simulink model "ExecutionTiming"  (R2014b)
settings: Solver=ode3  StartTime=0.0  StopTime=60  RelTol=1e-3
libraries: LegIK x6, BeagleBoneBlackCom x2, ServoCommand x2, MainController x1, Coord_BodyToLeg x1, TriggerSystem x1
settings Model: SimulationMode=processor-in-the-loop (pil)  Creator=dan  LastModifiedBy=Sebastian
settings SolverCC: InsertRTBMode=Never (minimum delay)
settings DataIOCC: SaveOutput=off  InspectSignalLogs=on  SaveTime=off
settings OptimizationCC: ExpressionDepthLimit=2147483647  OptimizeModelRefInitCode=on  LifeSpan=1  MaxStackSize=64
settings DebuggingCC: UnderspecifiedInitializationDetection=Classic  MergeDetectMultiDrivingBlocksExec=none  SignalResolutionControl=TryResolveAllWithWarning  MultiTaskDSMMsg=warning  MultiTaskCondExecSysMsg=none  ParameterPrecisionLossMsg=none  FcnCallInpInsideContextMsg=UseLocalSettings  UnconnectedInputMsg=none  UnconnectedOutputMsg=none  StateNameClashWarn=warning
settings HardwareCC: ProdLargestAtomicInteger=Long  ProdLargestAtomicFloat=Double  ProdEndianess=LittleEndian  ProdHWDeviceType=ARM Compatible->ARM Cortex  TargetBitPerChar=16  TargetBitPerInt=16  TargetBitPerPointer=16  TargetLargestAtomicInteger=Integer  TargetIntDivRoundTo=Zero  TargetEndianess=LittleEndian  TargetWordSize=16  TargetHWDeviceType=Texas Instruments->C2000
settings RTWCC: SystemTargetFile=ert.tlc  TemplateMakefile=ert_default_tmf  Description=Embedded Coder  ProcessScript=ert_make_rtw_hook  Toolchain=Linaro Toolchain v4.8  BuildConfiguration=Specify  CodeExecutionProfiling=on  CodeExecutionProfileVariable=executionProfile99  CodeProfilingSaveOptions=AllData  IncludeERTFirstTime=on
settings CodeAppCC: IgnoreCustomStorageClasses=off  CustomSymbolStrType=$N$R$M  InternalIdentifier=Classic
settings ERTTargetCC: CodeReplacementLibrary=ARM Cortex-A  MatFileLogging=on  SupportNonInlinedSFcns=on  SupportVariableSizeSignals=on

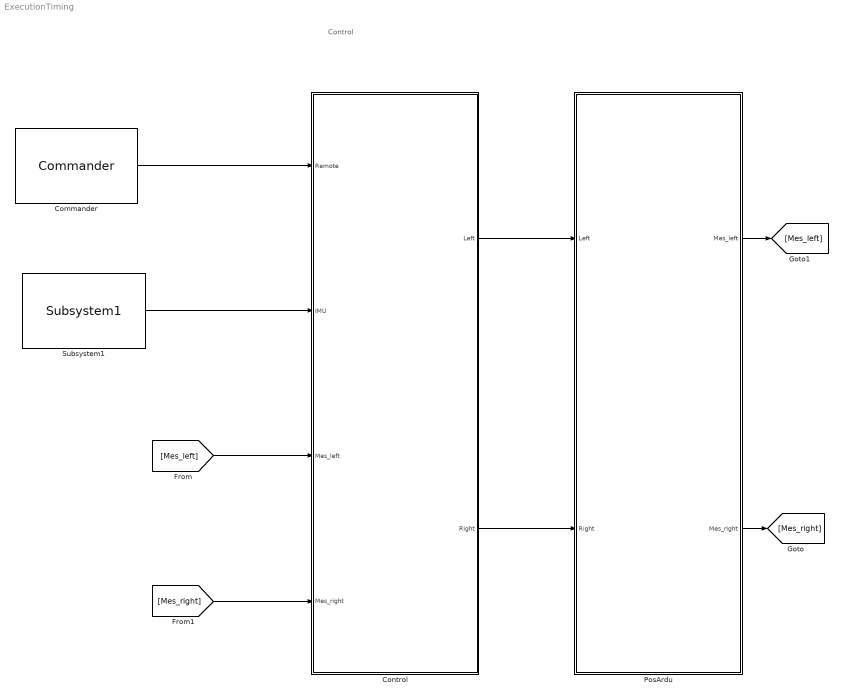
== system ExecutionTiming ==
  note: Control
  Commander : BeagleBoneBlackCom/Commander  portNbr=Uart 2
  Control : Subsystem  TreatAsAtomicUnit=on
  PosArdu : Subsystem  TreatAsAtomicUnit=on
  Subsystem1 : BeagleBoneBlackCom/Subsystem1  Priority=3  SystemSampleTime=-1
  wires:
  [Mes_right] -> Control/4(Mes_right)
  [Mes_left] -> Control/3(Mes_left)
  PosArdu/2(Mes_right) -> [Mes_right]
  PosArdu/1(Mes_left) -> [Mes_left]
  Control/1(Left) -> PosArdu/1(Left)
  Control/2(Right) -> PosArdu/2(Right)
  Commander/1 -> Control/1(Remote)
  Subsystem1/1 -> Control/2(IMU)

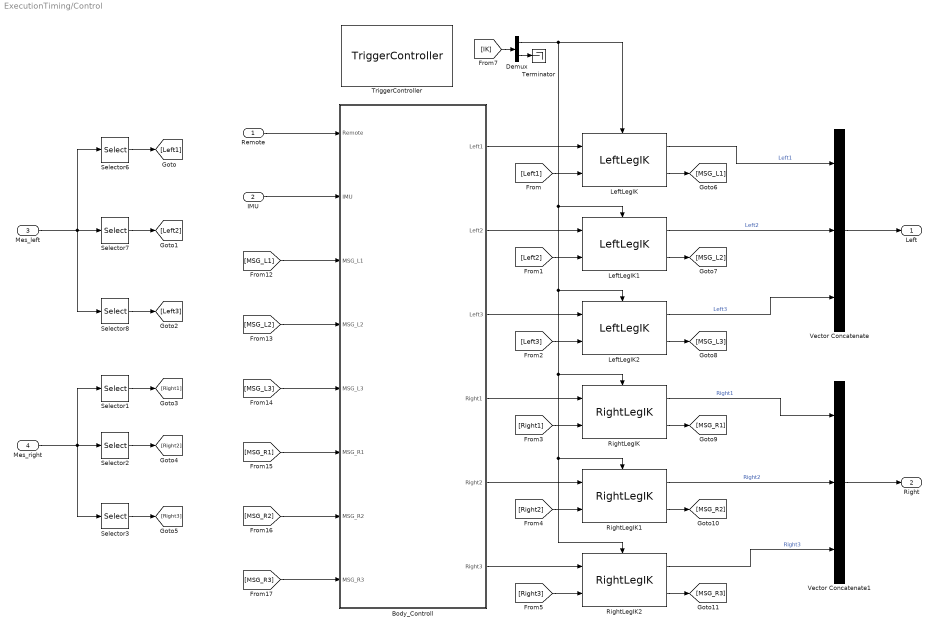
== system ExecutionTiming/Control ==
  Remote : Inport  OutDataTypeStr=Bus: Command
  IMU : Inport  Port=2
  Mes_left : Inport  Port=3  OutDataTypeStr=Bus: Leg_mes
  Mes_right : Inport  Port=4  OutDataTypeStr=Bus: Leg_mes
  Body_Controll : Subsystem
  Demux : Demux  Outputs=2
  LeftLegIK : LegIK/LeftLegIK  ID1=1  ID2=3  ID3=5
  LeftLegIK1 : LegIK/LeftLegIK  ID1=13  ID2=15  ID3=17
  LeftLegIK2 : LegIK/LeftLegIK  ID1=7  ID2=9  ID3=11
  RightLegIK : LegIK/RightLegIK  ID1=2  ID2=4  ID3=6
  RightLegIK1 : LegIK/RightLegIK  ID1=14  ID2=16  ID3=18
  RightLegIK2 : LegIK/RightLegIK  ID1=8  ID2=10  ID3=12
  Selector1 : Selector  IndexMode=Zero-based  InputPortWidth=3  Indices=0
  Selector2 : Selector  IndexMode=Zero-based  InputPortWidth=3
  Selector3 : Selector  IndexMode=Zero-based  InputPortWidth=3  Indices=2
  Selector6 : Selector  IndexMode=Zero-based  InputPortWidth=3  Indices=0
  Selector7 : Selector  IndexMode=Zero-based  InputPortWidth=3
  Selector8 : Selector  IndexMode=Zero-based  InputPortWidth=3  Indices=2
  Terminator : Terminator
  TriggerController : TriggerSystem/TriggerController  f=40
  Vector Concatenate : Concatenate  NumInputs=3  ConcatenateDimension=2
  Vector Concatenate1 : Concatenate  NumInputs=3  ConcatenateDimension=2
  Left : Outport  OutDataTypeStr=Bus: Leg_ref
  Right : Outport  Port=2  OutDataTypeStr=Bus: Leg_ref
  wires:
  Body_Controll/2(Left2) -> LeftLegIK1/1
  Body_Controll/1(Left1) -> LeftLegIK/1
  Body_Controll/3(Left3) -> LeftLegIK2/1
  Body_Controll/5(Right2) -> RightLegIK1/1
  Body_Controll/4(Right1) -> RightLegIK/1
  Body_Controll/6(Right3) -> RightLegIK2/1
  Remote/1 -> Body_Controll/1(Remote)
  [Left3] -> LeftLegIK2/2
  [Right1] -> RightLegIK/2
  RightLegIK/2 -> [MSG_R1]
  [MSG_R3] -> Body_Controll/8(MSG_R3)
  [MSG_R2] -> Body_Controll/7(MSG_R2)
  [MSG_R1] -> Body_Controll/6(MSG_R1)
  [MSG_L3] -> Body_Controll/5(MSG_L3)
  [MSG_L2] -> Body_Controll/4(MSG_L2)
  [MSG_L1] -> Body_Controll/3(MSG_L1)
  RightLegIK2/2 -> [MSG_R3]
  LeftLegIK2/2 -> [MSG_L3]
  RightLegIK1/2 -> [MSG_R2]
  LeftLegIK1/2 -> [MSG_L2]
  LeftLegIK/2 -> [MSG_L1]
  [Right2] -> RightLegIK1/2
  IMU/1 -> Body_Controll/2(IMU)
  [Right3] -> RightLegIK2/2
  [Left1] -> LeftLegIK/2
  [Left2] -> LeftLegIK1/2
  LeftLegIK2/1 -> Vector Concatenate/3  "Left3"
  LeftLegIK1/1 -> Vector Concatenate/2  "Left2"
  LeftLegIK/1 -> Vector Concatenate/1  "Left1"
  Vector Concatenate/1 -> Left/1
  RightLegIK/1 -> Vector Concatenate1/1  "Right1"
  RightLegIK1/1 -> Vector Concatenate1/2  "Right2"
  RightLegIK2/1 -> Vector Concatenate1/3  "Right3"
  Vector Concatenate1/1 -> Right/1
  Mes_left/1 -> Selector6/1, Selector7/1, Selector8/1
  Selector6/1 -> [Left1]
  Selector7/1 -> [Left2]
  Selector8/1 -> [Left3]
  Mes_right/1 -> Selector3/1, Selector2/1, Selector1/1
  Selector1/1 -> [Right1]
  Selector2/1 -> [Right2]
  Selector3/1 -> [Right3]
  Demux/1 -> RightLegIK1/Trigger, RightLegIK2/Trigger, RightLegIK/Trigger, LeftLegIK2/Trigger, LeftLegIK1/Trigger, LeftLegIK/Trigger
  [IK] -> Demux/1
  Demux/2 -> Terminator/1

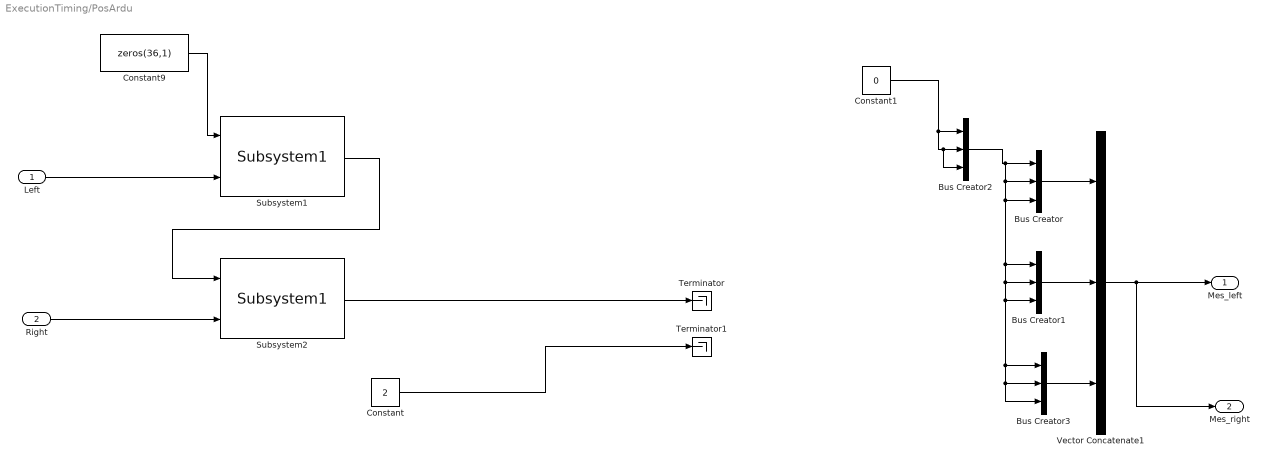
== system ExecutionTiming/PosArdu ==
  Left : Inport
  Right : Inport  Port=2
  Bus Creator : BusCreator  Inputs=3  OutDataTypeStr=Bus: Leg_mes  NonVirtualBus=on
  Bus Creator1 : BusCreator  Inputs=3  OutDataTypeStr=Bus: Leg_mes  NonVirtualBus=on
  Bus Creator2 : BusCreator  Inputs=3  OutDataTypeStr=Bus: Mes_servo  NonVirtualBus=on
      settings: InheritFromInputs=off
  Bus Creator3 : BusCreator  Inputs=3  OutDataTypeStr=Bus: Leg_mes  NonVirtualBus=on
  Constant : Constant  Value=2  OutDataTypeStr=uint8
  Constant1 : Constant  Value=0
  Constant9 : Constant  Value=zeros(36,1)  OutDataTypeStr=uint8  SampleTime=-1
  Subsystem1 : ServoCommand/Subsystem1
  Subsystem2 : ServoCommand/Subsystem1
  Terminator : Terminator
  Terminator1 : Terminator
  Vector Concatenate1 : Concatenate  NumInputs=3  ConcatenateDimension=2
  Mes_left : Outport
  Mes_right : Outport  Port=2
  wires:
  Subsystem1/1 -> Subsystem2/1
  Constant9/1 -> Subsystem1/1
  Bus Creator2/1 -> Bus Creator3/3, Bus Creator3/2, Bus Creator3/1, Bus Creator1/3, Bus Creator1/2, Bus Creator1/1, Bus Creator/3, Bus Creator/2, Bus Creator/1
  Constant1/1 -> Bus Creator2/3, Bus Creator2/2, Bus Creator2/1
  Bus Creator/1 -> Vector Concatenate1/1
  Bus Creator1/1 -> Vector Concatenate1/2
  Bus Creator3/1 -> Vector Concatenate1/3
  Vector Concatenate1/1 -> Mes_right/1, Mes_left/1
  Subsystem2/1 -> Terminator/1
  Constant/1 -> Terminator1/1
  Left/1 -> Subsystem1/2
  Right/1 -> Subsystem2/2

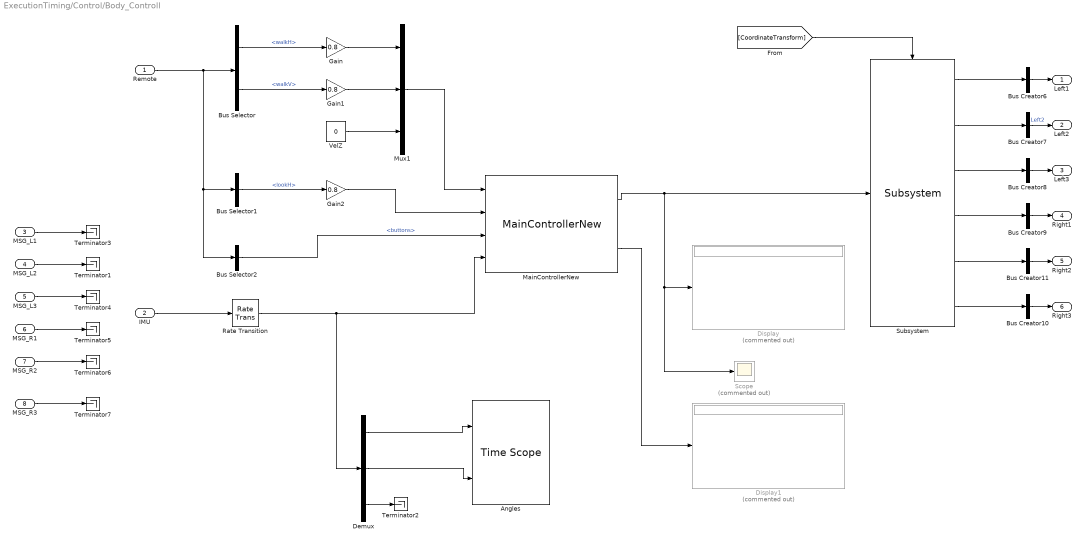
== system ExecutionTiming/Control/Body_Controll ==
  Remote : Inport  OutDataTypeStr=Bus: Command
  IMU : Inport  Port=2
  MSG_L1 : Inport  Port=3
  MSG_L2 : Inport  Port=4
  MSG_L3 : Inport  Port=5
  MSG_R1 : Inport  Port=6
  MSG_R2 : Inport  Port=7
  MSG_R3 : Inport  Port=8
  Angles : TimeScope  DefaultConfigurationName=spbscopes.TimeScopeBlockCfg  NumInputPorts=2
  Bus Creator{6..11} (6 alike) : BusCreator  Inputs=1  OutDataTypeStr=Bus: Leg_data
      settings: InheritFromInputs=off
  Bus Selector : BusSelector  OutputSignals=walkH,walkV
  Bus Selector1 : BusSelector  OutputSignals=lookH
  Bus Selector2 : BusSelector  OutputSignals=buttons
  Demux : Demux  Outputs=3
  Display : Display  Commented=on
  Display1 : Display  Commented=on
  Gain : Gain  Gain=0.8  OutDataTypeStr=double
  Gain1 : Gain  Gain=0.8  OutDataTypeStr=double
  Gain2 : Gain  Gain=0.8  OutDataTypeStr=double
  MainControllerNew : MainController/MainControllerNew
  Mux1 : Mux  Inputs=3
  Rate Transition : RateTransition  Deterministic=off  OutPortSampleTimeMultiple=0.5  OutPortSampleTime=0.0125
  Scope : Scope  Commented=on
      settings: YMin=-300  YMax=400  SaveName=ScopeData5
  Subsystem : Coord_BodyToLeg/Subsystem
  Terminator{1..7} (7 alike) : Terminator
  VelZ : Constant  Value=0  OutDataTypeStr=double  SampleTime=-1
  Left1 : Outport  OutDataTypeStr=Bus: Leg_data
  Left2 : Outport  Port=2  OutDataTypeStr=Bus: Leg_data
  Left3 : Outport  Port=3  OutDataTypeStr=Bus: Leg_data
  Right1 : Outport  Port=4  OutDataTypeStr=Bus: Leg_data
  Right2 : Outport  Port=5  OutDataTypeStr=Bus: Leg_data
  Right3 : Outport  Port=6  OutDataTypeStr=Bus: Leg_data
  wires:
  MSG_R3/1 -> Terminator7/1
  MSG_L1/1 -> Terminator3/1
  MSG_L2/1 -> Terminator1/1
  MSG_L3/1 -> Terminator4/1
  MSG_R1/1 -> Terminator5/1
  MSG_R2/1 -> Terminator6/1
  Subsystem/1 -> Bus Creator6/1
  Subsystem/2 -> Bus Creator7/1
  Subsystem/3 -> Bus Creator8/1
  Subsystem/4 -> Bus Creator9/1
  Subsystem/5 -> Bus Creator11/1
  Subsystem/6 -> Bus Creator10/1
  Bus Creator10/1 -> Right3/1
  Bus Creator11/1 -> Right2/1
  Bus Creator9/1 -> Right1/1
  Bus Creator8/1 -> Left3/1
  Bus Creator7/1 -> Left2/1  "Left2"
  Bus Creator6/1 -> Left1/1
  VelZ/1 -> Mux1/3
  Mux1/1 -> MainControllerNew/1
  MainControllerNew/1 -> Subsystem/1, Scope/1, Display/1
  MainControllerNew/2 -> Display1/1
  Bus Selector/1 -> Gain/1  "<walkH>"
  Bus Selector/2 -> Gain1/1  "<walkV>"
  Gain/1 -> Mux1/1
  Bus Selector1/1 -> Gain2/1  "<lookH>"
  Gain1/1 -> Mux1/2
  Remote/1 -> Bus Selector/1, Bus Selector2/1, Bus Selector1/1
  Bus Selector2/1 -> MainControllerNew/3  "<buttons>"
  Demux/1 -> Angles/1
  Demux/2 -> Angles/2
  [CoordinateTransform] -> Subsystem/Trigger
  Gain2/1 -> MainControllerNew/2
  IMU/1 -> Rate Transition/1
  Demux/3 -> Terminator2/1
  Rate Transition/1 -> Demux/1, MainControllerNew/4
